simulink model "sldemo_engine"  (R2024a)
settings: Solver=ode45  StartTime=0.0  StopTime=9.9  RelTol=1e-3  AbsTol=1e-6
Description:
  | Modeling Engine Timing Using Triggered Subsystems
  | 
  | This example shows how to model of a four-cylinder spark ignition engine
  | and shows Simulink(R) capabilities to model an internal combustion
  | engine from the throttle to the crankshaft output. We used well-defined
  | physical principles supplemented, where appropriate, with empirical
  | relationships that describe the systems dynamic behavior without
  | introducing unnecessary complexity.
settings Model: Creator=The MathWorks, Inc.  LastModifiedBy=uditpant
settings SolverCC: AutoScaleAbsTol=off  AlgebraicLoopSolver=TrustRegion
settings DataIOCC: ExternalInput=[]  InitialState=[]  SaveFormat=Array  SaveOutput=off  SaveTime=off  ReturnWorkspaceOutputs=off  StateSaveName=x  TimeSaveName=t  OutputSaveName=y  SignalLoggingName=sldemo_engine_output
settings OptimizationCC: BlockReduction=off  ExpressionDepthLimit=2147483647  InitFltsAndDblsToZero=on  LifeSpan=inf  BufferReusableBoundary=off
settings DebuggingCC: SaveWithParameterizedLinksMsg=none  SignalResolutionControl=TryResolveAllWithWarning  MultiTaskDSMMsg=warning  MultiTaskCondExecSysMsg=none  SigSpecEnsureSampleTimeMsg=none  IntegerOverflowMsg=none  FcnCallInpInsideContextMsg=warning  UnconnectedInputMsg=warning  UnconnectedOutputMsg=warning  UnconnectedLineMsg=warning  BusObjectLabelMismatch=none  StateNameClashWarn=warning  SFUnexpectedBacktrackingDiag=warning  SFNoUnconditionalDefaultTransitionDiag=warning  SFExecutionAtInitializationDiag=none  IntegerSaturationMsg=none  ArithmeticOperatorsInVariantConditions=warning
settings HardwareCC: ProdBitPerPointer=32  ProdBitPerSizeT=32  ProdBitPerPtrDiffT=32  ProdLargestAtomicFloat=None  ProdIntDivRoundTo=Undefined  ProdEndianess=Unspecified  ProdWordSize=32  ProdHWDeviceType=32-bit Generic
settings ModelReferenceCC: EnableRefExpFcnMdlSchedulingChecks=on  PropagateSignalLabelsOutOfModel=off
settings SFSimCC: SimUseLocalCustomCode=off  CustomCodeUndefinedFunction=UseInterfaceOnly
settings RTWCC: RTWUseLocalCustomCode=off  GPUComputeCapability=3.5
settings CodeAppCC: StateflowObjectComments=on
settings GRTTargetCC: TargetFcnLib=ansi_tfl_tmw.mat  TargetLangStandard=C89/C90 (ANSI)  CombineOutputUpdateFcns=off  GRTInterface=on
settings ConfigComp: CovMetricSettings=d  CovSaveCumulativeToWorkspaceVar=on  CovSaveSingleToWorkspaceVar=on  CovExternalEMLEnable=off

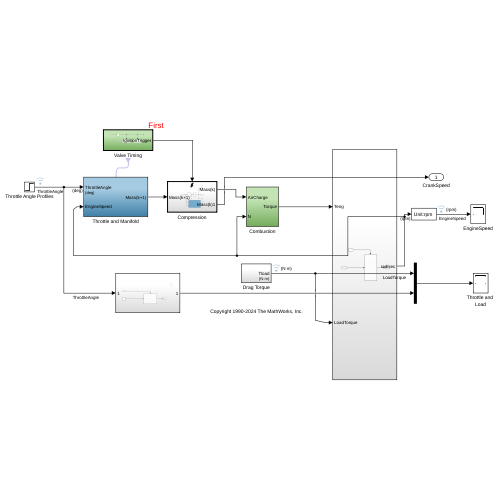
[thumbnail: Simulink's stored preview of the top-level diagram]
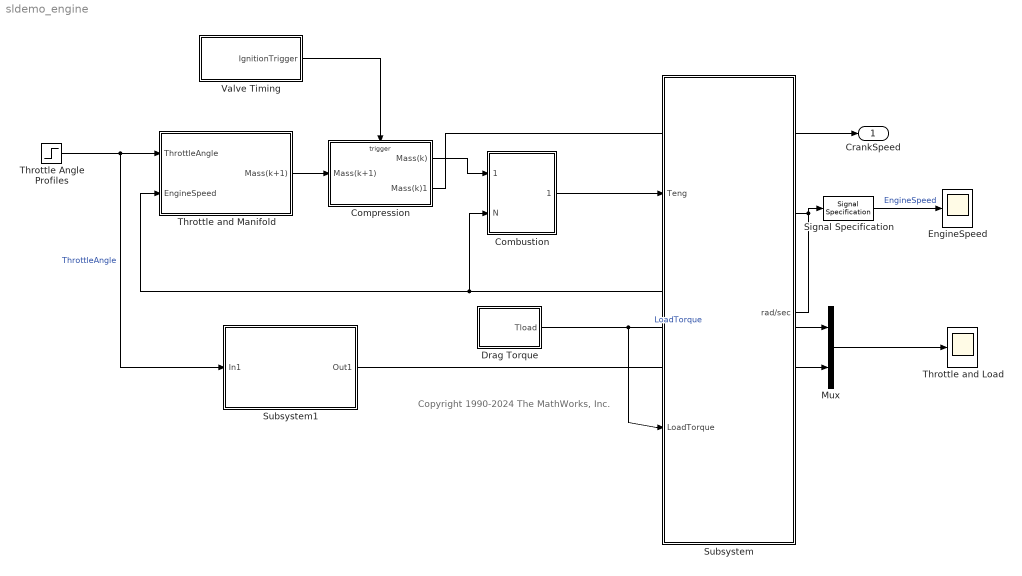
== system sldemo_engine ==
  note: Copyright 1990-2024 The MathWorks, Inc.
  Combustion : Subsystem
  Compression : Subsystem  TreatAsAtomicUnit=on
  Drag Torque : Subsystem
  EngineSpeed : Scope
  Mux : Mux  Inputs=2
  Signal Specification : SignalSpecification  Unit=rpm
  Subsystem : Subsystem
  Subsystem1 : Subsystem
  "Throttle Angle Profiles " : Step  Time=5  Before=8.973  After=11.93  SampleTime=0
  Throttle and Load : Scope
  Throttle and Manifold : Subsystem
  Valve Timing : Subsystem  ExecutionOrder=First  TreatAsAtomicUnit=on
  CrankSpeed : Outport  InitialOutput=0  VectorParamsAs1DForOutWhenUnconnected=off
  wires:
  Valve Timing/1(IgnitionTrigger) -> Compression/Trigger
  Throttle and Manifold/1(Mass(k+1)) -> Compression/1(Mass(k+1))
  Mux/1 -> Throttle and Load/1
  Compression/1(Mass(k)) -> Combustion/1(AirCharge)
  "Throttle Angle Profiles "/1 -> Throttle and Manifold/1(ThrottleAngle), Subsystem1/1(In1)  "ThrottleAngle"
  Drag Torque/1(Tload) -> Subsystem/2(LoadTorque), Mux/1  "LoadTorque"
  Signal Specification/1 -> EngineSpeed/1  "EngineSpeed"
  Compression/2(Mass(k)1) -> CrankSpeed/1
  Subsystem/1(rad/sec) -> Combustion/2(N), Throttle and Manifold/2(EngineSpeed), Signal Specification/1
  Combustion/1(Torque) -> Subsystem/1(Teng)
  Subsystem1/1(Out1) -> Mux/2

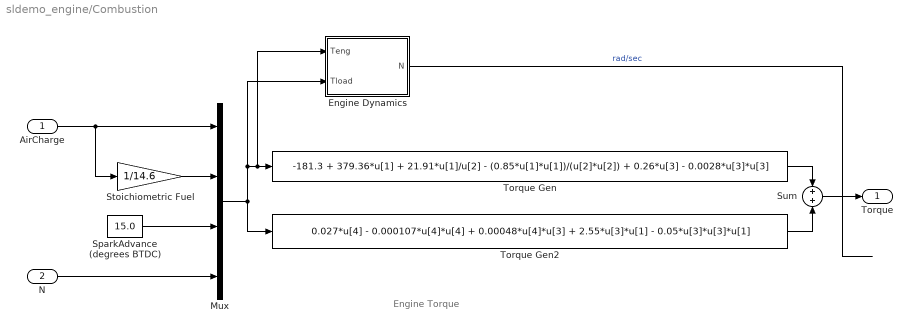
== system sldemo_engine/Combustion ==
  note: Engine Torque
  AirCharge : Inport
  N : Inport  Port=2
  Engine Dynamics : Subsystem
  Mux : Mux
  SparkAdvance (degrees BTDC) : Constant  Value=15.0
  Stoichiometric Fuel : Gain  Gain=1/14.6  SaturateOnIntegerOverflow=on  OutDataTypeStr=Inherit: Same as input  ParamDataTypeStr=Inherit: Same as input
  Sum : Sum  InputSameDT=on  SaturateOnIntegerOverflow=on  OutDataTypeStr=Inherit: Same as first input
  Torque Gen : Fcn  Expr=-181.3 + 379.36*u[1] + 21.91*u[1]/u[2] - (0.85*u[1]*u[1])/(u[2]*u[2]) + 0.26*u[3] - 0.0028*u[3]*u[3]
  Torque Gen2 : Fcn  Expr=0.027*u[4] - 0.000107*u[4]*u[4] + 0.00048*u[4]*u[3] + 2.55*u[3]*u[1] - 0.05*u[3]*u[3]*u[1]
  Torque : Outport  InitialOutput=0  VectorParamsAs1DForOutWhenUnconnected=off
  wires:
  Sum/1 -> Torque/1
  Torque Gen/1 -> Sum/1
  Torque Gen2/1 -> Sum/2
  Mux/1 -> Engine Dynamics/2(Tload), Engine Dynamics/1(Teng), Torque Gen/1, Torque Gen2/1
  AirCharge/1 -> Mux/1, Stoichiometric Fuel/1
  N/1 -> Mux/4
  SparkAdvance (degrees BTDC)/1 -> Mux/3
  Stoichiometric Fuel/1 -> Mux/2
  Engine Dynamics/1(N) -> ?  "rad/sec"

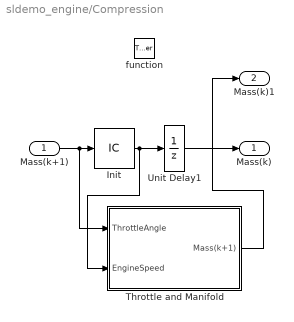
== system sldemo_engine/Compression ==
  Mass(k+1) : Inport
  function : TriggerPort  VariantControl=(inherit)  InitialTriggerSignalState=zero
  Init : InitialCondition  Value=0.152
  Throttle and Manifold : Subsystem
  Unit Delay1 : UnitDelay  InitialCondition=0.152  SampleTime=-1  HasFrameUpgradeWarning=on
  Mass(k) : Outport  InitialOutput=0.152  VectorParamsAs1DForOutWhenUnconnected=off
  Mass(k)1 : Outport  Port=2  InitialOutput=0.152  VectorParamsAs1DForOutWhenUnconnected=off
  wires:
  Unit Delay1/1 -> Mass(k)/1
  Init/1 -> Throttle and Manifold/2(EngineSpeed), Unit Delay1/1
  Mass(k+1)/1 -> Throttle and Manifold/1(ThrottleAngle), Init/1
  Throttle and Manifold/1(Mass(k+1)) -> Mass(k)1/1

== system sldemo_engine/Drag Torque ==
  note: Disturbances
  note: Torque
  Step : Step  Time=2  Before=25  After=20  SampleTime=0
  Step1 : Step  Time=8  After=5  SampleTime=0
  Subtract : Sum  Inputs=+-
  Tload : Outport  Unit=N*m  InitialOutput=0  VectorParamsAs1DForOutWhenUnconnected=off
  wires:
  Subtract/1 -> Tload/1
  Step/1 -> Subtract/1
  Step1/1 -> Subtract/2

== system sldemo_engine/Subsystem ==
  Teng : Inport
  LoadTorque : Inport  Port=2
  Triggered Subsystem : Subsystem  TreatAsAtomicUnit=on
  rad/sec : Outport
  wires:
  Triggered Subsystem/1(Out1) -> rad/sec/1  "rad/sec"
  Teng/1 -> Triggered Subsystem/Trigger
  LoadTorque/1 -> Triggered Subsystem/1(LoadTorque)

== system sldemo_engine/Subsystem1 ==
  In1 : Inport
  Callback Button : CustomCallbackButton  Configuration="{\"components\":[{\"name\":\"BackgroundImageComponent\",\"settings\":{\"image\":{\"size\":[0,0],\"src\":\"default\",\"srcOrientation\":\"Right\"},\"position\":[0,0,1,1]}},{\"name\":\"ButtonStateComponent\",\"settings\":{\"buttonType\":\"momentary\",\"clickFcn\":\"showExample(\\\"simulink_automotive\\/ModelingEngineTimingUsingTriggeredSubsystemsExample\\\")\",\"onValue\":1,\"position\":[0,0,1,1],\"pressDelay\":\"500\",\"pressFcn\":\"\",\"repeatInterval\":\"0\",\"states\":[{\"horizontalAlignment\":\"center\",\"image\":{\"position\":[0,0,1,1],\"size\":[1,1],\"src\":\"default\",\"srcOrientation\":\"Right\"},\"label\":{\"color\":[0.01176470588,0.01176470588,0.01176470588,1],\"icon\":{\"size\":[0,0],\"src\":\"default\",\"srcOrientation\":\"Right\"},\"iconPlacement\":\"left\",\"opacity\":1,\"show\":true,\"text\":{\"content\":\"?\",\"font\":\"Helvetica\",\"fontSize\":12}},\"labelOffset\":[0,0],\"verticalAlignment\":\"middle\"},{\"horizontalAlignment\":\"center\",\"image\":{\"position\":[0,0,1,1],\"size\":[1,1],\"src\":\"default\",\"srcOrientation\":\"Right\"},\"label\":{\"color\":[0.01176470588,0.01176470588,0.01176470588,1],\"icon\":{\"size\":[0,0],\"src\":\"default\",\"srcOrientation\":\"Right\"},\"iconPlacement\":\"left\",\"opacity\":1,\"show\":true,\"text\":{\"content\":\"?\",\"font\":\"Helvetica\",\"fontSize\":12}},\"labelOffset\":[0,0],\"verticalAlignment\":\"middle\"},{\"horizontalAlignment\":\"center\",\"image\":{\"position\":[0,0,1,1],\"size\":[1,1],\"src\":\"default\",\"srcOrientation\":\"Right\"},\"label\":{\"color\":[0.01176470588,0.01176470588,0.01176470588,1],\"icon\":{\"size\":[0,0],\"src\":\"default\",\"srcOrientation\":\"Right\"},\"iconPlacement\":\"left\",\"opacity\":1,\"show\":true,\"text\":{\"content\":\"?\",\"font\":\"Helvetica\",\"fontSize\":12}},\"labelOffset\":[0,0],\"verticalAlignment\":\"middle\"},{\"horizontalAlignment\":\"center\",\"image\":{\"position\":[0,0,1,1],\"size\":[1,1],\"src\":\"default\",\"srcOrientation\":\"Right\"},\"label\":{\"color\":[0.01176470588,0.01176470588,0.01176470588,1],\"icon\":{\"size\":[0,0],\"src\":\"default\",\"srcOrientation\":\"Right\"},\"iconPlacement\":\"left\",\"opacity\":1,\"show\":true,\"text\":{\"content\":\"?\",\"font\":\"Helvetica\",\"fontSize\":12}},\"labelOffset\":[0,0],\"verticalAlignment\":\"middle\"}]}},{\"name\":\"ForegroundImageComponent\",\"settings\":{\"image\":{\"size\":[0,0],\"src\":\"default\",\"srcOrientation\":\"Right\"},\"isForeground\":1,\"position\":[0,0,1,1]}}],\"settings\":{\"BindingType\":\"standalone\",\"backgroundColor\":[244,244,244,1],\"backgroundOffset\":0.2,\"backgroundOpacity\":1,\"fixedAspectRatio\":\"off\",\"foregroundColor\":[0.01176470588,0.01176470588,0.01176470588,1],\"migratedFromLegacy\":true,\"useBackgroundColor\":true,\"variant\":\"callback\",\"version\":\"R2023a\"},\"type\":\"Button\"}"  CustomBackgroundColor="{\"color\":[0.9568627451,0.9568627451,0.9568627451],\"show\":true}"
  Constant : Constant  Value=42
  Subsystem : Subsystem
  Out1 : Outport
  wires:
  In1/1 -> Subsystem/Enable
  Subsystem/1(Out1) -> Out1/1
  Constant/1 -> Subsystem/1(In1)

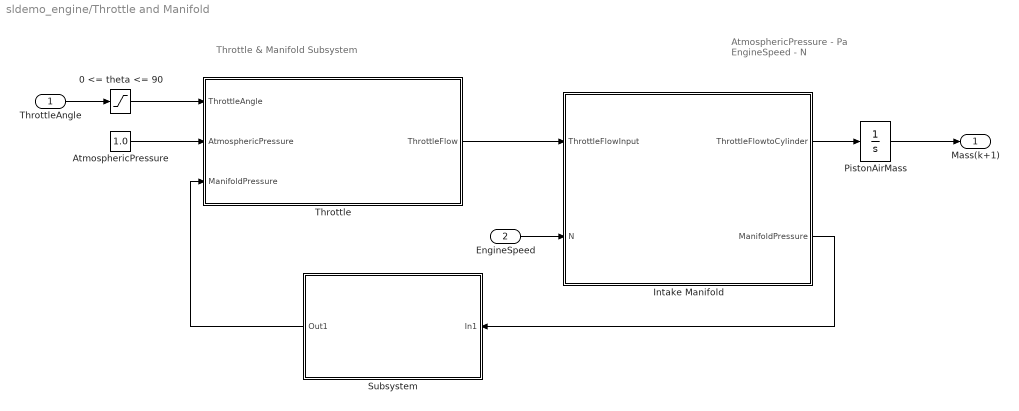
== system sldemo_engine/Throttle and Manifold ==
  note: AtmosphericPressure - Pa
      | EngineSpeed - N
  note: Throttle & Manifold Subsystem
  ThrottleAngle : Inport  Unit=deg
  EngineSpeed : Inport  Port=2
  0 <= theta <= 90 : Saturate  UpperLimit=90  LowerLimit=0
  AtmosphericPressure : Constant  Value=1.0
  Intake Manifold : Subsystem
  PistonAirMass : Integrator
  Subsystem : Subsystem
  Throttle : Subsystem
  Mass(k+1) : Outport  InitialOutput=0  VectorParamsAs1DForOutWhenUnconnected=off
  wires:
  0 <= theta <= 90/1 -> Throttle/1(ThrottleAngle)
  ThrottleAngle/1 -> 0 <= theta <= 90/1
  Throttle/1(ThrottleFlow) -> Intake Manifold/1(ThrottleFlowInput)
  EngineSpeed/1 -> Intake Manifold/2(N)
  AtmosphericPressure/1 -> Throttle/2("AtmosphericPressure ")
  Intake Manifold/1("ThrottleFlowtoCylinder ") -> PistonAirMass/1
  PistonAirMass/1 -> Mass(k+1)/1
  Intake Manifold/2(ManifoldPressure) -> Subsystem/1(In1)
  Subsystem/1(Out1) -> Throttle/3(ManifoldPressure)

== system sldemo_engine/Valve Timing ==
  Reset Crank Angle on Rising Edge : Subsystem  TreatAsAtomicUnit=on
  Reset Piston Air Mass on Falling Edge : Subsystem  TreatAsAtomicUnit=on
  State Reader : StateReader
  TDC and BDC Detection : HitCross  HitCrossingOffset=pi  HitCrossingDirection=rising
  IgnitionTrigger : Outport
  wires:
  State Reader/1 -> TDC and BDC Detection/1
  TDC and BDC Detection/1 -> IgnitionTrigger/1, Reset Piston Air Mass on Falling Edge/Trigger, Reset Crank Angle on Rising Edge/Trigger

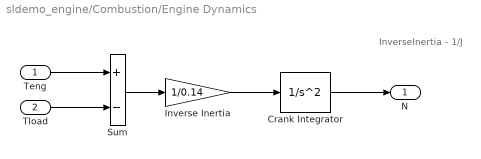
== system sldemo_engine/Combustion/Engine Dynamics ==
  note: InverseInertia - 1/J
  Teng : Inport
  Tload : Inport  Port=2
  Crank Integrator : SecondOrderIntegrator  ICX=0  StateNameX='CrankAngle'  ICDXDT=209.48  StateNameDXDT='CrankAngleVelocity'  ShowOutput=dxdt
  Inverse Inertia : Gain  Gain=1/0.14  SaturateOnIntegerOverflow=on  OutDataTypeStr=Inherit: Same as input  ParamDataTypeStr=Inherit: Same as input
  Sum : Sum  Inputs=+-  InputSameDT=on  SaturateOnIntegerOverflow=on  OutDataTypeStr=Inherit: Same as first input
  N : Outport  Unit=rad/sec  InitialOutput=0  VectorParamsAs1DForOutWhenUnconnected=off
  wires:
  Tload/1 -> Sum/2
  Teng/1 -> Sum/1
  Sum/1 -> Inverse Inertia/1
  Inverse Inertia/1 -> Crank Integrator/1
  Crank Integrator/1 -> N/1

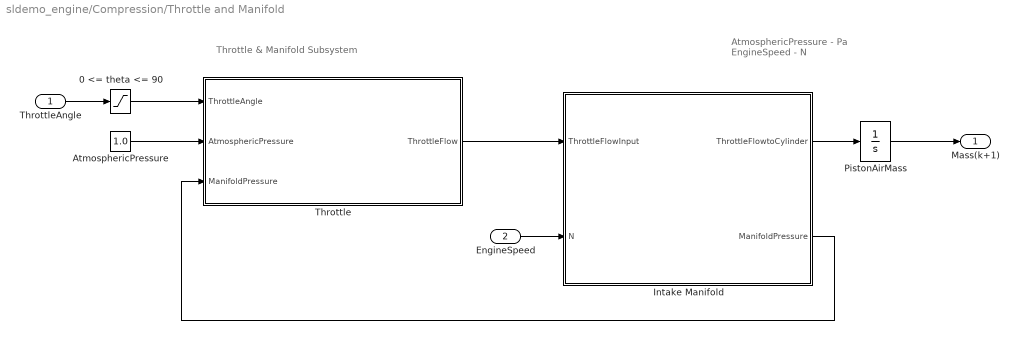
== system sldemo_engine/Compression/Throttle and Manifold ==
  note: AtmosphericPressure - Pa
      | EngineSpeed - N
  note: Throttle & Manifold Subsystem
  ThrottleAngle : Inport  Unit=deg
  EngineSpeed : Inport  Port=2
  0 <= theta <= 90 : Saturate  UpperLimit=90  LowerLimit=0
  AtmosphericPressure : Constant  Value=1.0
  Intake Manifold : Subsystem
  PistonAirMass : Integrator
  Throttle : Subsystem
  Mass(k+1) : Outport  InitialOutput=0  VectorParamsAs1DForOutWhenUnconnected=off
  wires:
  0 <= theta <= 90/1 -> Throttle/1(ThrottleAngle)
  ThrottleAngle/1 -> 0 <= theta <= 90/1
  Throttle/1(ThrottleFlow) -> Intake Manifold/1(ThrottleFlowInput)
  EngineSpeed/1 -> Intake Manifold/2(N)
  Intake Manifold/2(ManifoldPressure) -> Throttle/3(ManifoldPressure)
  AtmosphericPressure/1 -> Throttle/2("AtmosphericPressure ")
  Intake Manifold/1("ThrottleFlowtoCylinder ") -> PistonAirMass/1
  PistonAirMass/1 -> Mass(k+1)/1

== system sldemo_engine/Subsystem/Triggered Subsystem ==
  LoadTorque : Inport
  Trigger : TriggerPort  VariantControl=(inherit)
  Out1 : Outport
  wires:
  LoadTorque/1 -> Out1/1

== system sldemo_engine/Subsystem1/Subsystem ==
  In1 : Inport
  Enable : EnablePort
  Gain : Gain
  Out1 : Outport
  wires:
  In1/1 -> Gain/1
  Gain/1 -> Out1/1

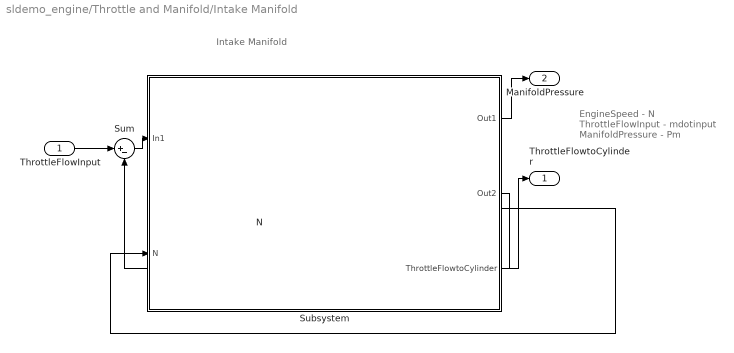
== system sldemo_engine/Throttle and Manifold/Intake Manifold ==
  note: EngineSpeed - N
      | ThrottleFlowInput - mdotinput
      | ManifoldPressure - Pm
  note: Intake Manifold
  ThrottleFlowInput : Inport
  N : Inport  Port=2  Unit=rad/sec
  Subsystem : Subsystem
  Sum : Sum  Inputs=|+-  InputSameDT=on  SaturateOnIntegerOverflow=on  OutDataTypeStr=Inherit: Same as first input
  "ThrottleFlowtoCylinder " : Outport  Unit=g/s  InitialOutput=0  VectorParamsAs1DForOutWhenUnconnected=off
  ManifoldPressure : Outport  Port=2  InitialOutput=0  VectorParamsAs1DForOutWhenUnconnected=off
  wires:
  ThrottleFlowInput/1 -> Sum/1
  Sum/1 -> Subsystem/1(In1)
  N/1 -> Subsystem/2(N)
  Subsystem/1(Out1) -> ManifoldPressure/1
  Subsystem/2(Out2) -> Sum/2
  Subsystem/3("ThrottleFlowtoCylinder ") -> "ThrottleFlowtoCylinder "/1

== system sldemo_engine/Throttle and Manifold/Subsystem ==
  In1 : Inport
  rad/sec to rpm : UnitConversion
  Out1 : Outport
  wires:
  rad/sec to rpm/1 -> Out1/1
  In1/1 -> rad/sec to rpm/1

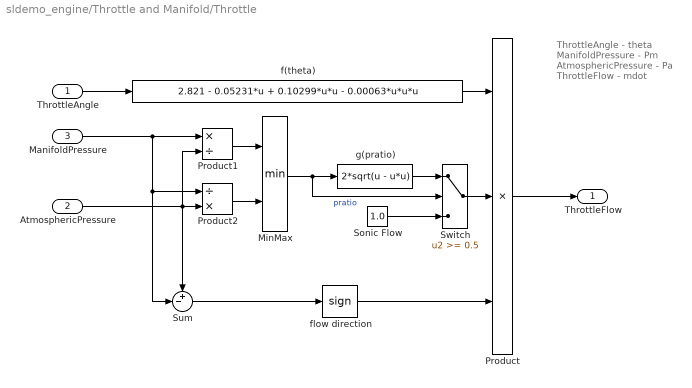
== system sldemo_engine/Throttle and Manifold/Throttle ==
  note: ThrottleAngle - theta
      | ManifoldPressure - Pm
      | AtmosphericPressure - Pa
      | ThrottleFlow - mdot
  ThrottleAngle : Inport  Unit=deg
  "AtmosphericPressure " : Inport  Port=2  Unit=bar
  ManifoldPressure : Inport  Port=3  Unit=bar
  MinMax : MinMax  Inputs=2  InputSameDT=on  SaturateOnIntegerOverflow=on
  Product : Product  Inputs=3  InputSameDT=on  RndMeth=Zero  SaturateOnIntegerOverflow=on  OutDataTypeStr=Inherit: Same as first input
  Product1 : Product  Inputs=*/  InputSameDT=on  RndMeth=Zero  SaturateOnIntegerOverflow=on  OutDataTypeStr=Inherit: Same as first input
  Product2 : Product  Inputs=/*  InputSameDT=on  RndMeth=Zero  SaturateOnIntegerOverflow=on  OutDataTypeStr=Inherit: Same as first input
  "Sonic Flow " : Constant  Value=1.0
  Sum : Sum  Inputs=+-|  InputSameDT=on  SaturateOnIntegerOverflow=on  OutDataTypeStr=Inherit: Same as first input
  Switch : Switch  Threshold=0.5
  f(theta) : Fcn  Expr=2.821 - 0.05231*u + 0.10299*u*u - 0.00063*u*u*u
  flow direction : Signum
  g(pratio) : Fcn  Expr=2*sqrt(u - u*u)
  ThrottleFlow : Outport  Unit=g/s  InitialOutput=0  VectorParamsAs1DForOutWhenUnconnected=off
  wires:
  ManifoldPressure/1 -> Sum/2, Product2/1, Product1/1
  Product2/1 -> MinMax/2
  Product1/1 -> MinMax/1
  "AtmosphericPressure "/1 -> Product1/2, Sum/1, Product2/2
  g(pratio)/1 -> Switch/1
  "Sonic Flow "/1 -> Switch/3
  Switch/1 -> Product/2
  flow direction/1 -> Product/3
  Sum/1 -> flow direction/1
  MinMax/1 -> Switch/2, g(pratio)/1  "pratio"
  ThrottleAngle/1 -> f(theta)/1
  Product/1 -> ThrottleFlow/1
  f(theta)/1 -> Product/1

== system sldemo_engine/Valve Timing/Reset Crank Angle on Rising Edge ==
  function : TriggerPort  VariantControl=(inherit)  InitialTriggerSignalState=zero
  Constant : Constant  Value=0
  State Writer : StateWriter
  wires:
  Constant/1 -> State Writer/1

== system sldemo_engine/Valve Timing/Reset Piston Air Mass on Falling Edge ==
  function : TriggerPort  TriggerType=falling  VariantControl=(inherit)  InitialTriggerSignalState=zero
  Constant1 : Constant  Value=0
  State Writer1 : StateWriter  StateOwnerBlock=../../../Throttle and Manifold/PistonAirMass
  wires:
  Constant1/1 -> State Writer1/1

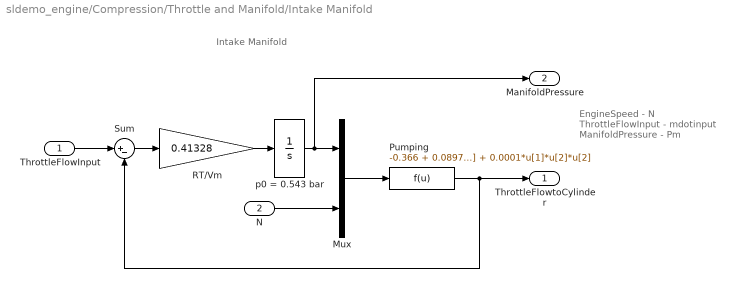
== system sldemo_engine/Compression/Throttle and Manifold/Intake Manifold ==
  note: EngineSpeed - N
      | ThrottleFlowInput - mdotinput
      | ManifoldPressure - Pm
  note: Intake Manifold
  ThrottleFlowInput : Inport
  N : Inport  Port=2  Unit=rad/sec
  Mux : Mux  Inputs=2
  Pumping : Fcn  Expr=-0.366 + 0.08979*u[1]*u[2] - 0.0337*u[2]*u[1]*u[1] + 0.0001*u[1]*u[2]*u[2]
  RT/Vm : Gain  Gain=0.41328  SaturateOnIntegerOverflow=on  OutDataTypeStr=Inherit: Same as input  ParamDataTypeStr=Inherit: Same as input
  Sum : Sum  Inputs=|+-  InputSameDT=on  SaturateOnIntegerOverflow=on  OutDataTypeStr=Inherit: Same as first input
  p0 = 0.543 bar : Integrator  InitialCondition=.543
  "ThrottleFlowtoCylinder " : Outport  Unit=g/s  InitialOutput=0  VectorParamsAs1DForOutWhenUnconnected=off
  ManifoldPressure : Outport  Port=2  InitialOutput=0  VectorParamsAs1DForOutWhenUnconnected=off
  wires:
  ThrottleFlowInput/1 -> Sum/1
  RT/Vm/1 -> p0 = 0.543 bar/1
  N/1 -> Mux/2
  Mux/1 -> Pumping/1
  p0 = 0.543 bar/1 -> Mux/1, ManifoldPressure/1
  Sum/1 -> RT/Vm/1
  Pumping/1 -> Sum/2, "ThrottleFlowtoCylinder "/1

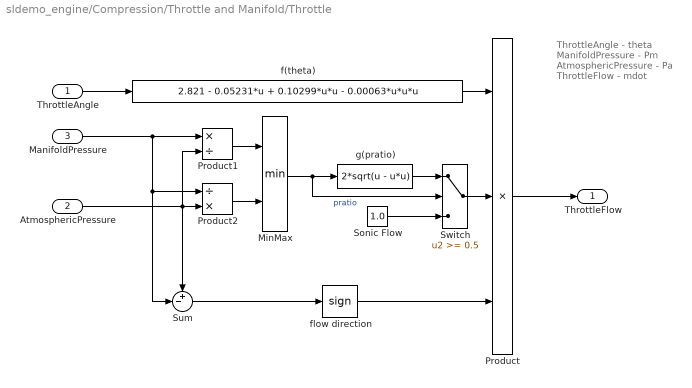
== system sldemo_engine/Compression/Throttle and Manifold/Throttle ==
  note: ThrottleAngle - theta
      | ManifoldPressure - Pm
      | AtmosphericPressure - Pa
      | ThrottleFlow - mdot
  ThrottleAngle : Inport  Unit=deg
  "AtmosphericPressure " : Inport  Port=2  Unit=bar
  ManifoldPressure : Inport  Port=3  Unit=bar
  MinMax : MinMax  Inputs=2  InputSameDT=on  SaturateOnIntegerOverflow=on
  Product : Product  Inputs=3  InputSameDT=on  RndMeth=Zero  SaturateOnIntegerOverflow=on  OutDataTypeStr=Inherit: Same as first input
  Product1 : Product  Inputs=*/  InputSameDT=on  RndMeth=Zero  SaturateOnIntegerOverflow=on  OutDataTypeStr=Inherit: Same as first input
  Product2 : Product  Inputs=/*  InputSameDT=on  RndMeth=Zero  SaturateOnIntegerOverflow=on  OutDataTypeStr=Inherit: Same as first input
  "Sonic Flow " : Constant  Value=1.0
  Sum : Sum  Inputs=+-|  InputSameDT=on  SaturateOnIntegerOverflow=on  OutDataTypeStr=Inherit: Same as first input
  Switch : Switch  Threshold=0.5
  f(theta) : Fcn  Expr=2.821 - 0.05231*u + 0.10299*u*u - 0.00063*u*u*u
  flow direction : Signum
  g(pratio) : Fcn  Expr=2*sqrt(u - u*u)
  ThrottleFlow : Outport  Unit=g/s  InitialOutput=0  VectorParamsAs1DForOutWhenUnconnected=off
  wires:
  ManifoldPressure/1 -> Sum/2, Product2/1, Product1/1
  Product2/1 -> MinMax/2
  Product1/1 -> MinMax/1
  "AtmosphericPressure "/1 -> Product1/2, Sum/1, Product2/2
  g(pratio)/1 -> Switch/1
  "Sonic Flow "/1 -> Switch/3
  Switch/1 -> Product/2
  flow direction/1 -> Product/3
  Sum/1 -> flow direction/1
  MinMax/1 -> Switch/2, g(pratio)/1  "pratio"
  ThrottleAngle/1 -> f(theta)/1
  Product/1 -> ThrottleFlow/1
  f(theta)/1 -> Product/1

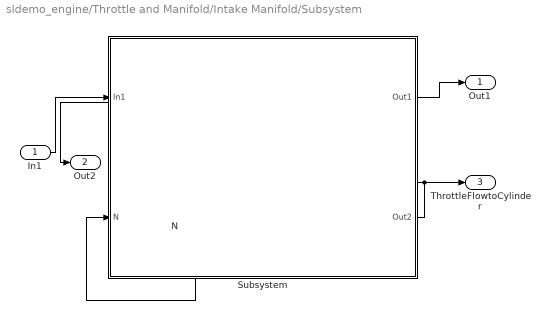
== system sldemo_engine/Throttle and Manifold/Intake Manifold/Subsystem ==
  In1 : Inport
  N : Inport  Port=2  Unit=rad/sec
  Subsystem : Subsystem
  Out1 : Outport
  Out2 : Outport  Port=2
  "ThrottleFlowtoCylinder " : Outport  Port=3  Unit=g/s  InitialOutput=0  VectorParamsAs1DForOutWhenUnconnected=off
  wires:
  Subsystem/2(Out2) -> Out2/1, "ThrottleFlowtoCylinder "/1
  In1/1 -> Subsystem/1(In1)
  N/1 -> Subsystem/2(N)
  Subsystem/1(Out1) -> Out1/1

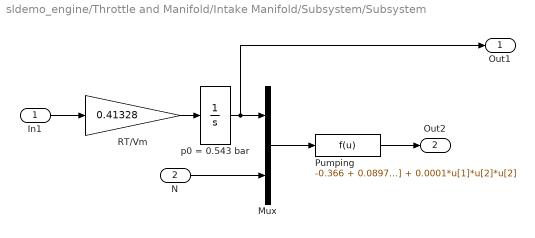
== system sldemo_engine/Throttle and Manifold/Intake Manifold/Subsystem/Subsystem ==
  In1 : Inport
  N : Inport  Port=2  Unit=rad/sec
  Mux : Mux  Inputs=2
  Pumping : Fcn  Expr=-0.366 + 0.08979*u[1]*u[2] - 0.0337*u[2]*u[1]*u[1] + 0.0001*u[1]*u[2]*u[2]
  RT/Vm : Gain  Gain=0.41328  SaturateOnIntegerOverflow=on  OutDataTypeStr=Inherit: Same as input  ParamDataTypeStr=Inherit: Same as input
  p0 = 0.543 bar : Integrator  InitialCondition=.543
  Out1 : Outport
  Out2 : Outport  Port=2
  wires:
  Mux/1 -> Pumping/1
  N/1 -> Mux/2
  RT/Vm/1 -> p0 = 0.543 bar/1
  p0 = 0.543 bar/1 -> Out1/1, Mux/1
  In1/1 -> RT/Vm/1
  Pumping/1 -> Out2/1
